simulink model "resonance_td"  (R2022a)
settings: Solver=VariableStepAuto  StartTime=0.0  StopTime=10.0  RelTol=1e-3
undefined symbols (not defined in the file): w0
settings Model: Creator=tstef  LastModifiedBy=tstef

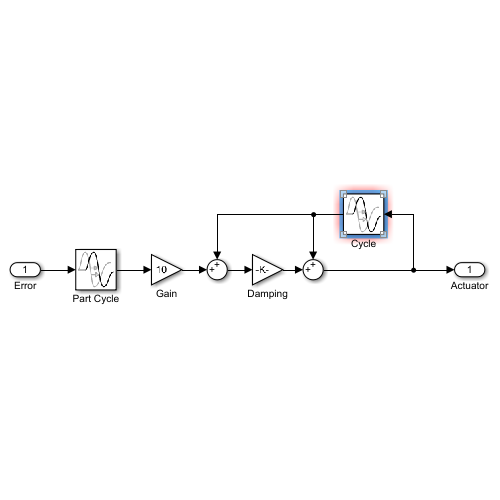
[thumbnail: Simulink's stored preview of the top-level diagram]
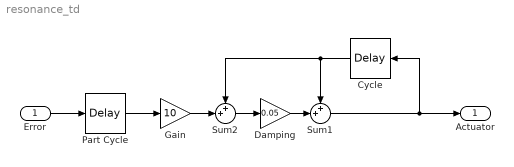
== system resonance_td ==
  Error : Inport
  Cycle : TransportDelay  DelayTime=2*pi/w0  PadeOrder=20
  Damping : Gain  Gain=0.05
  Gain : Gain  Gain=10
  Part Cycle : TransportDelay  DelayTime=0.09  PadeOrder=20
  Sum1 : Sum  Inputs=++|
  Sum2 : Sum  Inputs=++|
  Actuator : Outport
  wires:
  Error/1 -> Part Cycle/1
  Sum1/1 -> Cycle/1, Actuator/1
  Cycle/1 -> Sum2/1, Sum1/1
  Sum2/1 -> Damping/1
  Gain/1 -> Sum2/2
  Damping/1 -> Sum1/2
  Part Cycle/1 -> Gain/1
